simulink library "gnss_sdr_galileo_e1_tcp_connector_tracking_lib"  (Simulink 7.6)
settings: Solver=VariableStepDiscrete  StartTime=0.0  StopTime=10.0  RelTol=1e-3
undefined symbols (not defined in the file or in its folder): B_DLL, B_PLL, d_pdi_carr, d_pdi_code, k_DLL, k_PLL, magnitude, zeta_DLL, zeta_PLL
libraries: simulink x746, instrumentlib x2, dspindex x1
(part 5 of 5)

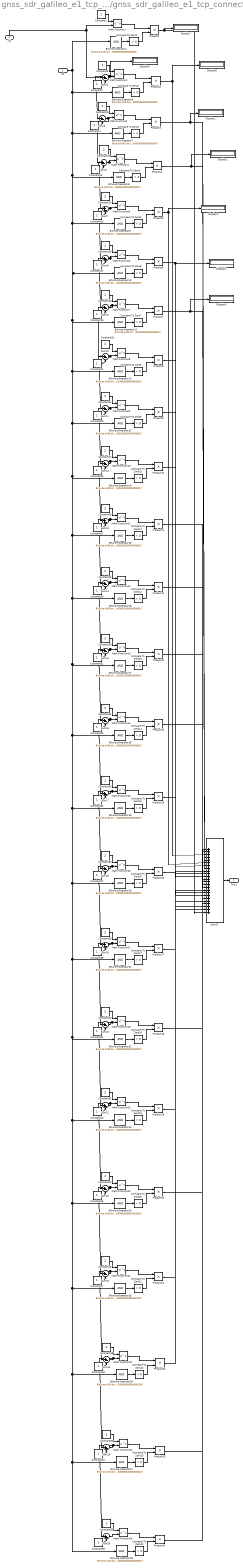
== system gnss_sdr_galileo_e1_tcp_connector_tracking_lib/gnss_sdr/gnss_sdr_galileo_e1_tcp_connector_tracking_rx/Subsystem6/hex2float/Subsystem ==
  In1 : Inport
  In2 : Inport  Port=2
  Bitwise Operator1 : simulink/Logic and Bit Operations/Bitwise Operator  logicop=AND  UseBitMask=on  BitMask=bin2dec('0100000000000000000000000')  BitMaskRealWorld=Stored Integer
  Bitwise Operator10 : simulink/Logic and Bit Operations/Bitwise Operator  logicop=AND  UseBitMask=on  BitMask=bin2dec('0000001000000000000000000')  BitMaskRealWorld=Stored Integer
  Bitwise Operator11 : simulink/Logic and Bit Operations/Bitwise Operator  logicop=AND  UseBitMask=on  BitMask=bin2dec('0000000100000000000000000')  BitMaskRealWorld=Stored Integer
  Bitwise Operator12 : simulink/Logic and Bit Operations/Bitwise Operator  logicop=AND  UseBitMask=on  BitMask=bin2dec('0000000010000000000000000')  BitMaskRealWorld=Stored Integer
  Bitwise Operator13 : simulink/Logic and Bit Operations/Bitwise Operator  logicop=AND  UseBitMask=on  BitMask=bin2dec('0000000001000000000000000')  BitMaskRealWorld=Stored Integer
  Bitwise Operator14 : simulink/Logic and Bit Operations/Bitwise Operator  logicop=AND  UseBitMask=on  BitMask=bin2dec('0000000000100000000000000')  BitMaskRealWorld=Stored Integer
  Bitwise Operator15 : simulink/Logic and Bit Operations/Bitwise Operator  logicop=AND  UseBitMask=on  BitMask=bin2dec('0000000000010000000000000')  BitMaskRealWorld=Stored Integer
  Bitwise Operator16 : simulink/Logic and Bit Operations/Bitwise Operator  logicop=AND  UseBitMask=on  BitMask=bin2dec('0000000000001000000000000')  BitMaskRealWorld=Stored Integer
  Bitwise Operator17 : simulink/Logic and Bit Operations/Bitwise Operator  logicop=AND  UseBitMask=on  BitMask=bin2dec('0000000000000100000000000')  BitMaskRealWorld=Stored Integer
  Bitwise Operator18 : simulink/Logic and Bit Operations/Bitwise Operator  logicop=AND  UseBitMask=on  BitMask=bin2dec('0000000000000010000000000')  BitMaskRealWorld=Stored Integer
  Bitwise Operator19 : simulink/Logic and Bit Operations/Bitwise Operator  logicop=AND  UseBitMask=on  BitMask=bin2dec('0000000000000001000000000')  BitMaskRealWorld=Stored Integer
  Bitwise Operator20 : simulink/Logic and Bit Operations/Bitwise Operator  logicop=AND  UseBitMask=on  BitMask=bin2dec('0000000000000000100000000')  BitMaskRealWorld=Stored Integer
  Bitwise Operator21 : simulink/Logic and Bit Operations/Bitwise Operator  logicop=AND  UseBitMask=on  BitMask=bin2dec('0000000000000000010000000')  BitMaskRealWorld=Stored Integer
  Bitwise Operator22 : simulink/Logic and Bit Operations/Bitwise Operator  logicop=AND  UseBitMask=on  BitMask=bin2dec('0000000000000000001000000')  BitMaskRealWorld=Stored Integer
  Bitwise Operator23 : simulink/Logic and Bit Operations/Bitwise Operator  logicop=AND  UseBitMask=on  BitMask=bin2dec('0000000000000000000100000')  BitMaskRealWorld=Stored Integer
  Bitwise Operator24 : simulink/Logic and Bit Operations/Bitwise Operator  logicop=AND  UseBitMask=on  BitMask=bin2dec('0000000000000000000010000')  BitMaskRealWorld=Stored Integer
  Bitwise Operator25 : simulink/Logic and Bit Operations/Bitwise Operator  logicop=AND  UseBitMask=on  BitMask=bin2dec('0000000000000000000001000')  BitMaskRealWorld=Stored Integer
  Bitwise Operator26 : simulink/Logic and Bit Operations/Bitwise Operator  logicop=AND  UseBitMask=on  BitMask=bin2dec('0000000000000000000000100')  BitMaskRealWorld=Stored Integer
  Bitwise Operator27 : simulink/Logic and Bit Operations/Bitwise Operator  logicop=AND  UseBitMask=on  BitMask=bin2dec('0000000000000000000000010')  BitMaskRealWorld=Stored Integer
  Bitwise Operator28 : simulink/Logic and Bit Operations/Bitwise Operator  logicop=AND  UseBitMask=on  BitMask=bin2dec('0000000000000000000000001')  BitMaskRealWorld=Stored Integer
  Bitwise Operator6 : simulink/Logic and Bit Operations/Bitwise Operator  logicop=AND  UseBitMask=on  BitMask=bin2dec('0010000000000000000000000')  BitMaskRealWorld=Stored Integer
  Bitwise Operator7 : simulink/Logic and Bit Operations/Bitwise Operator  logicop=AND  UseBitMask=on  BitMask=bin2dec('0001000000000000000000000')  BitMaskRealWorld=Stored Integer
  Bitwise Operator8 : simulink/Logic and Bit Operations/Bitwise Operator  logicop=AND  UseBitMask=on  BitMask=bin2dec('0000100000000000000000000')  BitMaskRealWorld=Stored Integer
  Bitwise Operator9 : simulink/Logic and Bit Operations/Bitwise Operator  logicop=AND  UseBitMask=on  BitMask=bin2dec('0000010000000000000000000')  BitMaskRealWorld=Stored Integer
  Compare To Zero{1..24} (24 alike) : simulink/Logic and Bit Operations/Compare To Zero  SystemSampleTime=-1  relop=>  LogicOutDataTypeMode=uint8  ZeroCross=off
  Constant{1,8,10,12,14,16,18,20,22,24,26,28,30,32,34,36,38,40,42,44,46,48,50,52} (24 alike) : Constant  Value=2
  Constant{2,11,13,15,17,19,21,23,25,27,29,31,33,35,37,39,41,43,45,47,49,51,53} (23 alike) : Constant
  Display{1..8} (8 alike) : Display
  Math Function{1..24} (24 alike) : Math  Operator=pow  SaturateOnIntegerOverflow=on
  Product{1..24} (24 alike) : Product  RndMeth=Zero
  Sum{1,5..26} (23 alike) : Sum  Inputs=|+-
  Sum27 : Sum  Inputs=|++++++++++++++++++++++++
  Out1 : Outport
  wires:
  Constant8/1 -> Math Function2/1
  Bitwise Operator6/1 -> Compare To Zero2/1
  Compare To Zero2/1 -> Product2/2
  Math Function2/1 -> Product2/1
  Constant10/1 -> Math Function3/1
  Bitwise Operator7/1 -> Compare To Zero3/1
  Compare To Zero3/1 -> Product3/2
  Math Function3/1 -> Product3/1
  Constant11/1 -> Sum5/2
  Sum5/1 -> Sum6/1, Math Function3/2
  Constant12/1 -> Math Function4/1
  Bitwise Operator8/1 -> Compare To Zero4/1
  Compare To Zero4/1 -> Product4/2
  Math Function4/1 -> Product4/1
  Constant13/1 -> Sum6/2
  Sum6/1 -> Sum7/1, Math Function4/2
  Constant14/1 -> Math Function5/1
  Bitwise Operator9/1 -> Compare To Zero5/1
  Compare To Zero5/1 -> Product5/2
  Math Function5/1 -> Product5/1
  Constant15/1 -> Sum7/2
  Sum7/1 -> Sum8/1, Math Function5/2
  Constant16/1 -> Math Function6/1
  Bitwise Operator10/1 -> Compare To Zero6/1
  Compare To Zero6/1 -> Product6/2
  Math Function6/1 -> Product6/1
  Constant17/1 -> Sum8/2
  Sum8/1 -> Sum9/1, Math Function6/2
  Constant18/1 -> Math Function7/1
  Bitwise Operator11/1 -> Compare To Zero7/1
  Compare To Zero7/1 -> Product7/2
  Math Function7/1 -> Product7/1
  Constant19/1 -> Sum9/2
  Sum9/1 -> Math Function7/2, Sum10/1
  Constant20/1 -> Math Function8/1
  Bitwise Operator12/1 -> Compare To Zero8/1
  Compare To Zero8/1 -> Product8/2
  Math Function8/1 -> Product8/1
  Constant21/1 -> Sum10/2
  Sum10/1 -> Math Function8/2, Sum11/1
  Constant22/1 -> Math Function9/1
  Bitwise Operator13/1 -> Compare To Zero9/1
  Compare To Zero9/1 -> Product9/2
  Math Function9/1 -> Product9/1
  Constant23/1 -> Sum11/2
  Sum11/1 -> Math Function9/2, Sum12/1
  Constant24/1 -> Math Function10/1
  Bitwise Operator14/1 -> Compare To Zero10/1
  Compare To Zero10/1 -> Product10/2
  Math Function10/1 -> Product10/1
  Constant25/1 -> Sum12/2
  Sum12/1 -> Math Function10/2, Sum13/1
  Constant26/1 -> Math Function11/1
  Bitwise Operator15/1 -> Compare To Zero11/1
  Compare To Zero11/1 -> Product11/2
  Math Function11/1 -> Product11/1
  Constant27/1 -> Sum13/2
  Sum13/1 -> Math Function11/2, Sum14/1
  Constant28/1 -> Math Function12/1
  Bitwise Operator16/1 -> Compare To Zero12/1
  Compare To Zero12/1 -> Product12/2
  Math Function12/1 -> Product12/1
  Constant29/1 -> Sum14/2
  Sum14/1 -> Math Function12/2, Sum15/1
  Constant30/1 -> Math Function13/1
  Bitwise Operator17/1 -> Compare To Zero13/1
  Compare To Zero13/1 -> Product13/2
  Math Function13/1 -> Product13/1
  Constant31/1 -> Sum15/2
  Sum15/1 -> Math Function13/2, Sum16/1
  Constant32/1 -> Math Function14/1
  Bitwise Operator18/1 -> Compare To Zero14/1
  Compare To Zero14/1 -> Product14/2
  Math Function14/1 -> Product14/1
  Constant33/1 -> Sum16/2
  Sum16/1 -> Math Function14/2, Sum17/1
  Constant34/1 -> Math Function15/1
  Bitwise Operator19/1 -> Compare To Zero15/1
  Compare To Zero15/1 -> Product15/2
  Math Function15/1 -> Product15/1
  Constant35/1 -> Sum17/2
  Sum17/1 -> Math Function15/2, Sum18/1
  Constant36/1 -> Math Function16/1
  Bitwise Operator20/1 -> Compare To Zero16/1
  Compare To Zero16/1 -> Product16/2
  Math Function16/1 -> Product16/1
  Constant37/1 -> Sum18/2
  Sum18/1 -> Math Function16/2, Sum19/1
  Constant38/1 -> Math Function17/1
  Bitwise Operator21/1 -> Compare To Zero17/1
  Compare To Zero17/1 -> Product17/2
  Math Function17/1 -> Product17/1
  Constant39/1 -> Sum19/2
  Sum19/1 -> Math Function17/2, Sum20/1
  Constant40/1 -> Math Function18/1
  Bitwise Operator22/1 -> Compare To Zero18/1
  Compare To Zero18/1 -> Product18/2
  Math Function18/1 -> Product18/1
  Constant41/1 -> Sum20/2
  Sum20/1 -> Math Function18/2, Sum21/1
  Constant42/1 -> Math Function19/1
  Bitwise Operator23/1 -> Compare To Zero19/1
  Compare To Zero19/1 -> Product19/2
  Math Function19/1 -> Product19/1
  Constant43/1 -> Sum21/2
  Sum21/1 -> Math Function19/2, Sum22/1
  Constant44/1 -> Math Function20/1
  Bitwise Operator24/1 -> Compare To Zero20/1
  Compare To Zero20/1 -> Product20/2
  Math Function20/1 -> Product20/1
  Constant45/1 -> Sum22/2
  Sum22/1 -> Math Function20/2, Sum23/1
  Constant46/1 -> Math Function21/1
  Bitwise Operator25/1 -> Compare To Zero21/1
  Compare To Zero21/1 -> Product21/2
  Math Function21/1 -> Product21/1
  Constant47/1 -> Sum23/2
  Sum23/1 -> Math Function21/2, Sum24/1
  Constant48/1 -> Math Function22/1
  Bitwise Operator26/1 -> Compare To Zero22/1
  Compare To Zero22/1 -> Product22/2
  Math Function22/1 -> Product22/1
  Constant49/1 -> Sum24/2
  Sum24/1 -> Math Function22/2, Sum25/1
  Constant50/1 -> Math Function23/1
  Bitwise Operator27/1 -> Compare To Zero23/1
  Compare To Zero23/1 -> Product23/2
  Math Function23/1 -> Product23/1
  Constant51/1 -> Sum25/2
  Sum25/1 -> Math Function23/2, Sum26/1
  Constant52/1 -> Math Function24/1
  Bitwise Operator28/1 -> Compare To Zero24/1
  Compare To Zero24/1 -> Product24/2
  Math Function24/1 -> Product24/1
  Constant53/1 -> Sum26/2
  Sum26/1 -> Math Function24/2
  Product2/1 -> Sum27/3, Display5/1
  Product3/1 -> Sum27/4, Display1/1
  Product4/1 -> Sum27/5, Display2/1
  Product5/1 -> Sum27/6, Display3/1
  Product6/1 -> Sum27/7, Display4/1
  Product7/1 -> Sum27/8, Display6/1
  Product8/1 -> Sum27/9
  Product9/1 -> Sum27/10
  Product10/1 -> Sum27/11
  Product11/1 -> Sum27/12
  Product12/1 -> Sum27/13
  Product13/1 -> Sum27/14
  Product14/1 -> Sum27/15
  Product15/1 -> Sum27/16
  Product16/1 -> Sum27/17
  Product17/1 -> Sum27/18
  Product18/1 -> Sum27/19
  Product19/1 -> Sum27/20
  Product20/1 -> Sum27/21
  Product21/1 -> Sum27/22
  Product22/1 -> Sum27/23
  Product23/1 -> Sum27/2
  Product24/1 -> Sum27/1
  In1/1 -> Math Function1/2, Sum1/1
  In2/1 -> Bitwise Operator6/1, Bitwise Operator7/1, Bitwise Operator8/1, Bitwise Operator9/1, Bitwise Operator10/1, Bitwise Operator11/1, Bitwise Operator12/1, Bitwise Operator13/1, Bitwise Operator14/1, Bitwise Operator15/1, Bitwise Operator16/1, Bitwise Operator17/1, Bitwise Operator18/1, Bitwise Operator19/1, Bitwise Operator20/1, Bitwise Operator21/1, Bitwise Operator22/1, Bitwise Operator23/1, Bitwise Operator24/1, Bitwise Operator25/1, Bitwise Operator26/1, Bitwise Operator27/1, Bitwise Operator28/1, Bitwise Operator1/1
  Sum27/1 -> Out1/1
  Constant1/1 -> Math Function1/1
  Bitwise Operator1/1 -> Compare To Zero1/1
  Compare To Zero1/1 -> Product1/2
  Math Function1/1 -> Product1/1
  Constant2/1 -> Sum1/2
  Sum1/1 -> Math Function2/2, Display8/1, Sum5/1
  Product1/1 -> Display7/1, Sum27/24

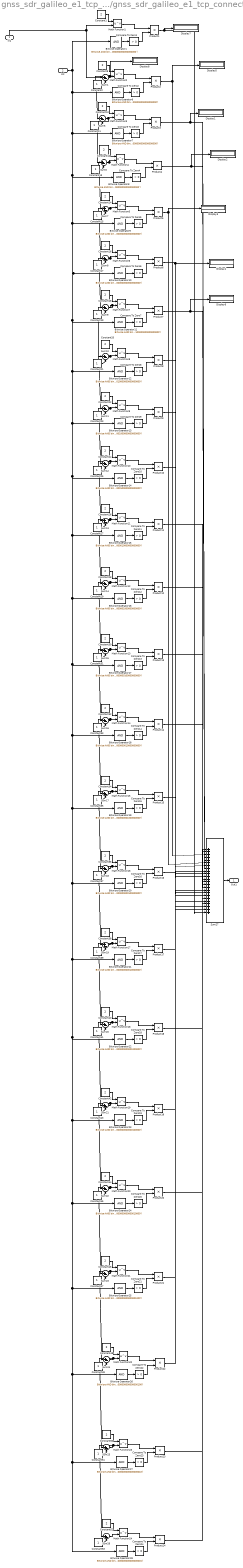
== system gnss_sdr_galileo_e1_tcp_connector_tracking_lib/gnss_sdr/gnss_sdr_galileo_e1_tcp_connector_tracking_rx/Subsystem7/hex2float/Subsystem ==
  In1 : Inport
  In2 : Inport  Port=2
  Bitwise Operator1 : simulink/Logic and Bit Operations/Bitwise Operator  logicop=AND  UseBitMask=on  BitMask=bin2dec('0100000000000000000000000')  BitMaskRealWorld=Stored Integer
  Bitwise Operator10 : simulink/Logic and Bit Operations/Bitwise Operator  logicop=AND  UseBitMask=on  BitMask=bin2dec('0000001000000000000000000')  BitMaskRealWorld=Stored Integer
  Bitwise Operator11 : simulink/Logic and Bit Operations/Bitwise Operator  logicop=AND  UseBitMask=on  BitMask=bin2dec('0000000100000000000000000')  BitMaskRealWorld=Stored Integer
  Bitwise Operator12 : simulink/Logic and Bit Operations/Bitwise Operator  logicop=AND  UseBitMask=on  BitMask=bin2dec('0000000010000000000000000')  BitMaskRealWorld=Stored Integer
  Bitwise Operator13 : simulink/Logic and Bit Operations/Bitwise Operator  logicop=AND  UseBitMask=on  BitMask=bin2dec('0000000001000000000000000')  BitMaskRealWorld=Stored Integer
  Bitwise Operator14 : simulink/Logic and Bit Operations/Bitwise Operator  logicop=AND  UseBitMask=on  BitMask=bin2dec('0000000000100000000000000')  BitMaskRealWorld=Stored Integer
  Bitwise Operator15 : simulink/Logic and Bit Operations/Bitwise Operator  logicop=AND  UseBitMask=on  BitMask=bin2dec('0000000000010000000000000')  BitMaskRealWorld=Stored Integer
  Bitwise Operator16 : simulink/Logic and Bit Operations/Bitwise Operator  logicop=AND  UseBitMask=on  BitMask=bin2dec('0000000000001000000000000')  BitMaskRealWorld=Stored Integer
  Bitwise Operator17 : simulink/Logic and Bit Operations/Bitwise Operator  logicop=AND  UseBitMask=on  BitMask=bin2dec('0000000000000100000000000')  BitMaskRealWorld=Stored Integer
  Bitwise Operator18 : simulink/Logic and Bit Operations/Bitwise Operator  logicop=AND  UseBitMask=on  BitMask=bin2dec('0000000000000010000000000')  BitMaskRealWorld=Stored Integer
  Bitwise Operator19 : simulink/Logic and Bit Operations/Bitwise Operator  logicop=AND  UseBitMask=on  BitMask=bin2dec('0000000000000001000000000')  BitMaskRealWorld=Stored Integer
  Bitwise Operator20 : simulink/Logic and Bit Operations/Bitwise Operator  logicop=AND  UseBitMask=on  BitMask=bin2dec('0000000000000000100000000')  BitMaskRealWorld=Stored Integer
  Bitwise Operator21 : simulink/Logic and Bit Operations/Bitwise Operator  logicop=AND  UseBitMask=on  BitMask=bin2dec('0000000000000000010000000')  BitMaskRealWorld=Stored Integer
  Bitwise Operator22 : simulink/Logic and Bit Operations/Bitwise Operator  logicop=AND  UseBitMask=on  BitMask=bin2dec('0000000000000000001000000')  BitMaskRealWorld=Stored Integer
  Bitwise Operator23 : simulink/Logic and Bit Operations/Bitwise Operator  logicop=AND  UseBitMask=on  BitMask=bin2dec('0000000000000000000100000')  BitMaskRealWorld=Stored Integer
  Bitwise Operator24 : simulink/Logic and Bit Operations/Bitwise Operator  logicop=AND  UseBitMask=on  BitMask=bin2dec('0000000000000000000010000')  BitMaskRealWorld=Stored Integer
  Bitwise Operator25 : simulink/Logic and Bit Operations/Bitwise Operator  logicop=AND  UseBitMask=on  BitMask=bin2dec('0000000000000000000001000')  BitMaskRealWorld=Stored Integer
  Bitwise Operator26 : simulink/Logic and Bit Operations/Bitwise Operator  logicop=AND  UseBitMask=on  BitMask=bin2dec('0000000000000000000000100')  BitMaskRealWorld=Stored Integer
  Bitwise Operator27 : simulink/Logic and Bit Operations/Bitwise Operator  logicop=AND  UseBitMask=on  BitMask=bin2dec('0000000000000000000000010')  BitMaskRealWorld=Stored Integer
  Bitwise Operator28 : simulink/Logic and Bit Operations/Bitwise Operator  logicop=AND  UseBitMask=on  BitMask=bin2dec('0000000000000000000000001')  BitMaskRealWorld=Stored Integer
  Bitwise Operator6 : simulink/Logic and Bit Operations/Bitwise Operator  logicop=AND  UseBitMask=on  BitMask=bin2dec('0010000000000000000000000')  BitMaskRealWorld=Stored Integer
  Bitwise Operator7 : simulink/Logic and Bit Operations/Bitwise Operator  logicop=AND  UseBitMask=on  BitMask=bin2dec('0001000000000000000000000')  BitMaskRealWorld=Stored Integer
  Bitwise Operator8 : simulink/Logic and Bit Operations/Bitwise Operator  logicop=AND  UseBitMask=on  BitMask=bin2dec('0000100000000000000000000')  BitMaskRealWorld=Stored Integer
  Bitwise Operator9 : simulink/Logic and Bit Operations/Bitwise Operator  logicop=AND  UseBitMask=on  BitMask=bin2dec('0000010000000000000000000')  BitMaskRealWorld=Stored Integer
  Compare To Zero{1..24} (24 alike) : simulink/Logic and Bit Operations/Compare To Zero  SystemSampleTime=-1  relop=>  LogicOutDataTypeMode=uint8  ZeroCross=off
  Constant{1,8,10,12,14,16,18,20,22,24,26,28,30,32,34,36,38,40,42,44,46,48,50,52} (24 alike) : Constant  Value=2
  Constant{2,11,13,15,17,19,21,23,25,27,29,31,33,35,37,39,41,43,45,47,49,51,53} (23 alike) : Constant
  Display{1..8} (8 alike) : Display
  Math Function{1..24} (24 alike) : Math  Operator=pow  SaturateOnIntegerOverflow=on
  Product{1..24} (24 alike) : Product  RndMeth=Zero
  Sum{1,5..26} (23 alike) : Sum  Inputs=|+-
  Sum27 : Sum  Inputs=|++++++++++++++++++++++++
  Out1 : Outport
  wires:
  Product1/1 -> Sum27/24, Display7/1
  Sum1/1 -> Sum5/1, Display8/1, Math Function2/2
  Constant2/1 -> Sum1/2
  Math Function1/1 -> Product1/1
  Compare To Zero1/1 -> Product1/2
  Bitwise Operator1/1 -> Compare To Zero1/1
  Constant1/1 -> Math Function1/1
  Sum27/1 -> Out1/1
  In2/1 -> Bitwise Operator1/1, Bitwise Operator28/1, Bitwise Operator27/1, Bitwise Operator26/1, Bitwise Operator25/1, Bitwise Operator24/1, Bitwise Operator23/1, Bitwise Operator22/1, Bitwise Operator21/1, Bitwise Operator20/1, Bitwise Operator19/1, Bitwise Operator18/1, Bitwise Operator17/1, Bitwise Operator16/1, Bitwise Operator15/1, Bitwise Operator14/1, Bitwise Operator13/1, Bitwise Operator12/1, Bitwise Operator11/1, Bitwise Operator10/1, Bitwise Operator9/1, Bitwise Operator8/1, Bitwise Operator7/1, Bitwise Operator6/1
  In1/1 -> Sum1/1, Math Function1/2
  Product24/1 -> Sum27/1
  Product23/1 -> Sum27/2
  Product22/1 -> Sum27/23
  Product21/1 -> Sum27/22
  Product20/1 -> Sum27/21
  Product19/1 -> Sum27/20
  Product18/1 -> Sum27/19
  Product17/1 -> Sum27/18
  Product16/1 -> Sum27/17
  Product15/1 -> Sum27/16
  Product14/1 -> Sum27/15
  Product13/1 -> Sum27/14
  Product12/1 -> Sum27/13
  Product11/1 -> Sum27/12
  Product10/1 -> Sum27/11
  Product9/1 -> Sum27/10
  Product8/1 -> Sum27/9
  Product7/1 -> Display6/1, Sum27/8
  Product6/1 -> Display4/1, Sum27/7
  Product5/1 -> Display3/1, Sum27/6
  Product4/1 -> Display2/1, Sum27/5
  Product3/1 -> Display1/1, Sum27/4
  Product2/1 -> Display5/1, Sum27/3
  Sum26/1 -> Math Function24/2
  Constant53/1 -> Sum26/2
  Math Function24/1 -> Product24/1
  Compare To Zero24/1 -> Product24/2
  Bitwise Operator28/1 -> Compare To Zero24/1
  Constant52/1 -> Math Function24/1
  Sum25/1 -> Sum26/1, Math Function23/2
  Constant51/1 -> Sum25/2
  Math Function23/1 -> Product23/1
  Compare To Zero23/1 -> Product23/2
  Bitwise Operator27/1 -> Compare To Zero23/1
  Constant50/1 -> Math Function23/1
  Sum24/1 -> Sum25/1, Math Function22/2
  Constant49/1 -> Sum24/2
  Math Function22/1 -> Product22/1
  Compare To Zero22/1 -> Product22/2
  Bitwise Operator26/1 -> Compare To Zero22/1
  Constant48/1 -> Math Function22/1
  Sum23/1 -> Sum24/1, Math Function21/2
  Constant47/1 -> Sum23/2
  Math Function21/1 -> Product21/1
  Compare To Zero21/1 -> Product21/2
  Bitwise Operator25/1 -> Compare To Zero21/1
  Constant46/1 -> Math Function21/1
  Sum22/1 -> Sum23/1, Math Function20/2
  Constant45/1 -> Sum22/2
  Math Function20/1 -> Product20/1
  Compare To Zero20/1 -> Product20/2
  Bitwise Operator24/1 -> Compare To Zero20/1
  Constant44/1 -> Math Function20/1
  Sum21/1 -> Sum22/1, Math Function19/2
  Constant43/1 -> Sum21/2
  Math Function19/1 -> Product19/1
  Compare To Zero19/1 -> Product19/2
  Bitwise Operator23/1 -> Compare To Zero19/1
  Constant42/1 -> Math Function19/1
  Sum20/1 -> Sum21/1, Math Function18/2
  Constant41/1 -> Sum20/2
  Math Function18/1 -> Product18/1
  Compare To Zero18/1 -> Product18/2
  Bitwise Operator22/1 -> Compare To Zero18/1
  Constant40/1 -> Math Function18/1
  Sum19/1 -> Sum20/1, Math Function17/2
  Constant39/1 -> Sum19/2
  Math Function17/1 -> Product17/1
  Compare To Zero17/1 -> Product17/2
  Bitwise Operator21/1 -> Compare To Zero17/1
  Constant38/1 -> Math Function17/1
  Sum18/1 -> Sum19/1, Math Function16/2
  Constant37/1 -> Sum18/2
  Math Function16/1 -> Product16/1
  Compare To Zero16/1 -> Product16/2
  Bitwise Operator20/1 -> Compare To Zero16/1
  Constant36/1 -> Math Function16/1
  Sum17/1 -> Sum18/1, Math Function15/2
  Constant35/1 -> Sum17/2
  Math Function15/1 -> Product15/1
  Compare To Zero15/1 -> Product15/2
  Bitwise Operator19/1 -> Compare To Zero15/1
  Constant34/1 -> Math Function15/1
  Sum16/1 -> Sum17/1, Math Function14/2
  Constant33/1 -> Sum16/2
  Math Function14/1 -> Product14/1
  Compare To Zero14/1 -> Product14/2
  Bitwise Operator18/1 -> Compare To Zero14/1
  Constant32/1 -> Math Function14/1
  Sum15/1 -> Sum16/1, Math Function13/2
  Constant31/1 -> Sum15/2
  Math Function13/1 -> Product13/1
  Compare To Zero13/1 -> Product13/2
  Bitwise Operator17/1 -> Compare To Zero13/1
  Constant30/1 -> Math Function13/1
  Sum14/1 -> Sum15/1, Math Function12/2
  Constant29/1 -> Sum14/2
  Math Function12/1 -> Product12/1
  Compare To Zero12/1 -> Product12/2
  Bitwise Operator16/1 -> Compare To Zero12/1
  Constant28/1 -> Math Function12/1
  Sum13/1 -> Sum14/1, Math Function11/2
  Constant27/1 -> Sum13/2
  Math Function11/1 -> Product11/1
  Compare To Zero11/1 -> Product11/2
  Bitwise Operator15/1 -> Compare To Zero11/1
  Constant26/1 -> Math Function11/1
  Sum12/1 -> Sum13/1, Math Function10/2
  Constant25/1 -> Sum12/2
  Math Function10/1 -> Product10/1
  Compare To Zero10/1 -> Product10/2
  Bitwise Operator14/1 -> Compare To Zero10/1
  Constant24/1 -> Math Function10/1
  Sum11/1 -> Sum12/1, Math Function9/2
  Constant23/1 -> Sum11/2
  Math Function9/1 -> Product9/1
  Compare To Zero9/1 -> Product9/2
  Bitwise Operator13/1 -> Compare To Zero9/1
  Constant22/1 -> Math Function9/1
  Sum10/1 -> Sum11/1, Math Function8/2
  Constant21/1 -> Sum10/2
  Math Function8/1 -> Product8/1
  Compare To Zero8/1 -> Product8/2
  Bitwise Operator12/1 -> Compare To Zero8/1
  Constant20/1 -> Math Function8/1
  Sum9/1 -> Sum10/1, Math Function7/2
  Constant19/1 -> Sum9/2
  Math Function7/1 -> Product7/1
  Compare To Zero7/1 -> Product7/2
  Bitwise Operator11/1 -> Compare To Zero7/1
  Constant18/1 -> Math Function7/1
  Sum8/1 -> Math Function6/2, Sum9/1
  Constant17/1 -> Sum8/2
  Math Function6/1 -> Product6/1
  Compare To Zero6/1 -> Product6/2
  Bitwise Operator10/1 -> Compare To Zero6/1
  Constant16/1 -> Math Function6/1
  Sum7/1 -> Math Function5/2, Sum8/1
  Constant15/1 -> Sum7/2
  Math Function5/1 -> Product5/1
  Compare To Zero5/1 -> Product5/2
  Bitwise Operator9/1 -> Compare To Zero5/1
  Constant14/1 -> Math Function5/1
  Sum6/1 -> Math Function4/2, Sum7/1
  Constant13/1 -> Sum6/2
  Math Function4/1 -> Product4/1
  Compare To Zero4/1 -> Product4/2
  Bitwise Operator8/1 -> Compare To Zero4/1
  Constant12/1 -> Math Function4/1
  Sum5/1 -> Math Function3/2, Sum6/1
  Constant11/1 -> Sum5/2
  Math Function3/1 -> Product3/1
  Compare To Zero3/1 -> Product3/2
  Bitwise Operator7/1 -> Compare To Zero3/1
  Constant10/1 -> Math Function3/1
  Math Function2/1 -> Product2/1
  Compare To Zero2/1 -> Product2/2
  Bitwise Operator6/1 -> Compare To Zero2/1
  Constant8/1 -> Math Function2/1

== system gnss_sdr_galileo_e1_tcp_connector_tracking_lib/gnss_sdr/gnss_sdr_galileo_e1_tcp_connector_tracking_rx/Subsystem8/hex2float/Subsystem ==
  In1 : Inport
  In2 : Inport  Port=2
  Bitwise Operator1 : simulink/Logic and Bit Operations/Bitwise Operator  logicop=AND  UseBitMask=on  BitMask=bin2dec('0100000000000000000000000')  BitMaskRealWorld=Stored Integer
  Bitwise Operator10 : simulink/Logic and Bit Operations/Bitwise Operator  logicop=AND  UseBitMask=on  BitMask=bin2dec('0000001000000000000000000')  BitMaskRealWorld=Stored Integer
  Bitwise Operator11 : simulink/Logic and Bit Operations/Bitwise Operator  logicop=AND  UseBitMask=on  BitMask=bin2dec('0000000100000000000000000')  BitMaskRealWorld=Stored Integer
  Bitwise Operator12 : simulink/Logic and Bit Operations/Bitwise Operator  logicop=AND  UseBitMask=on  BitMask=bin2dec('0000000010000000000000000')  BitMaskRealWorld=Stored Integer
  Bitwise Operator13 : simulink/Logic and Bit Operations/Bitwise Operator  logicop=AND  UseBitMask=on  BitMask=bin2dec('0000000001000000000000000')  BitMaskRealWorld=Stored Integer
  Bitwise Operator14 : simulink/Logic and Bit Operations/Bitwise Operator  logicop=AND  UseBitMask=on  BitMask=bin2dec('0000000000100000000000000')  BitMaskRealWorld=Stored Integer
  Bitwise Operator15 : simulink/Logic and Bit Operations/Bitwise Operator  logicop=AND  UseBitMask=on  BitMask=bin2dec('0000000000010000000000000')  BitMaskRealWorld=Stored Integer
  Bitwise Operator16 : simulink/Logic and Bit Operations/Bitwise Operator  logicop=AND  UseBitMask=on  BitMask=bin2dec('0000000000001000000000000')  BitMaskRealWorld=Stored Integer
  Bitwise Operator17 : simulink/Logic and Bit Operations/Bitwise Operator  logicop=AND  UseBitMask=on  BitMask=bin2dec('0000000000000100000000000')  BitMaskRealWorld=Stored Integer
  Bitwise Operator18 : simulink/Logic and Bit Operations/Bitwise Operator  logicop=AND  UseBitMask=on  BitMask=bin2dec('0000000000000010000000000')  BitMaskRealWorld=Stored Integer
  Bitwise Operator19 : simulink/Logic and Bit Operations/Bitwise Operator  logicop=AND  UseBitMask=on  BitMask=bin2dec('0000000000000001000000000')  BitMaskRealWorld=Stored Integer
  Bitwise Operator20 : simulink/Logic and Bit Operations/Bitwise Operator  logicop=AND  UseBitMask=on  BitMask=bin2dec('0000000000000000100000000')  BitMaskRealWorld=Stored Integer
  Bitwise Operator21 : simulink/Logic and Bit Operations/Bitwise Operator  logicop=AND  UseBitMask=on  BitMask=bin2dec('0000000000000000010000000')  BitMaskRealWorld=Stored Integer
  Bitwise Operator22 : simulink/Logic and Bit Operations/Bitwise Operator  logicop=AND  UseBitMask=on  BitMask=bin2dec('0000000000000000001000000')  BitMaskRealWorld=Stored Integer
  Bitwise Operator23 : simulink/Logic and Bit Operations/Bitwise Operator  logicop=AND  UseBitMask=on  BitMask=bin2dec('0000000000000000000100000')  BitMaskRealWorld=Stored Integer
  Bitwise Operator24 : simulink/Logic and Bit Operations/Bitwise Operator  logicop=AND  UseBitMask=on  BitMask=bin2dec('0000000000000000000010000')  BitMaskRealWorld=Stored Integer
  Bitwise Operator25 : simulink/Logic and Bit Operations/Bitwise Operator  logicop=AND  UseBitMask=on  BitMask=bin2dec('0000000000000000000001000')  BitMaskRealWorld=Stored Integer
  Bitwise Operator26 : simulink/Logic and Bit Operations/Bitwise Operator  logicop=AND  UseBitMask=on  BitMask=bin2dec('0000000000000000000000100')  BitMaskRealWorld=Stored Integer
  Bitwise Operator27 : simulink/Logic and Bit Operations/Bitwise Operator  logicop=AND  UseBitMask=on  BitMask=bin2dec('0000000000000000000000010')  BitMaskRealWorld=Stored Integer
  Bitwise Operator28 : simulink/Logic and Bit Operations/Bitwise Operator  logicop=AND  UseBitMask=on  BitMask=bin2dec('0000000000000000000000001')  BitMaskRealWorld=Stored Integer
  Bitwise Operator6 : simulink/Logic and Bit Operations/Bitwise Operator  logicop=AND  UseBitMask=on  BitMask=bin2dec('0010000000000000000000000')  BitMaskRealWorld=Stored Integer
  Bitwise Operator7 : simulink/Logic and Bit Operations/Bitwise Operator  logicop=AND  UseBitMask=on  BitMask=bin2dec('0001000000000000000000000')  BitMaskRealWorld=Stored Integer
  Bitwise Operator8 : simulink/Logic and Bit Operations/Bitwise Operator  logicop=AND  UseBitMask=on  BitMask=bin2dec('0000100000000000000000000')  BitMaskRealWorld=Stored Integer
  Bitwise Operator9 : simulink/Logic and Bit Operations/Bitwise Operator  logicop=AND  UseBitMask=on  BitMask=bin2dec('0000010000000000000000000')  BitMaskRealWorld=Stored Integer
  Compare To Zero{1..24} (24 alike) : simulink/Logic and Bit Operations/Compare To Zero  SystemSampleTime=-1  relop=>  LogicOutDataTypeMode=uint8  ZeroCross=off
  Constant{1,8,10,12,14,16,18,20,22,24,26,28,30,32,34,36,38,40,42,44,46,48,50,52} (24 alike) : Constant  Value=2
  Constant{2,11,13,15,17,19,21,23,25,27,29,31,33,35,37,39,41,43,45,47,49,51,53} (23 alike) : Constant
  Display{1..8} (8 alike) : Display
  Math Function{1..24} (24 alike) : Math  Operator=pow  SaturateOnIntegerOverflow=on
  Product{1..24} (24 alike) : Product  RndMeth=Zero
  Sum{1,5..26} (23 alike) : Sum  Inputs=|+-
  Sum27 : Sum  Inputs=|++++++++++++++++++++++++
  Out1 : Outport
  wires:
  Product1/1 -> Sum27/24, Display7/1
  Sum1/1 -> Sum5/1, Display8/1, Math Function2/2
  Constant2/1 -> Sum1/2
  Math Function1/1 -> Product1/1
  Compare To Zero1/1 -> Product1/2
  Bitwise Operator1/1 -> Compare To Zero1/1
  Constant1/1 -> Math Function1/1
  Sum27/1 -> Out1/1
  In2/1 -> Bitwise Operator1/1, Bitwise Operator28/1, Bitwise Operator27/1, Bitwise Operator26/1, Bitwise Operator25/1, Bitwise Operator24/1, Bitwise Operator23/1, Bitwise Operator22/1, Bitwise Operator21/1, Bitwise Operator20/1, Bitwise Operator19/1, Bitwise Operator18/1, Bitwise Operator17/1, Bitwise Operator16/1, Bitwise Operator15/1, Bitwise Operator14/1, Bitwise Operator13/1, Bitwise Operator12/1, Bitwise Operator11/1, Bitwise Operator10/1, Bitwise Operator9/1, Bitwise Operator8/1, Bitwise Operator7/1, Bitwise Operator6/1
  In1/1 -> Sum1/1, Math Function1/2
  Product24/1 -> Sum27/1
  Product23/1 -> Sum27/2
  Product22/1 -> Sum27/23
  Product21/1 -> Sum27/22
  Product20/1 -> Sum27/21
  Product19/1 -> Sum27/20
  Product18/1 -> Sum27/19
  Product17/1 -> Sum27/18
  Product16/1 -> Sum27/17
  Product15/1 -> Sum27/16
  Product14/1 -> Sum27/15
  Product13/1 -> Sum27/14
  Product12/1 -> Sum27/13
  Product11/1 -> Sum27/12
  Product10/1 -> Sum27/11
  Product9/1 -> Sum27/10
  Product8/1 -> Sum27/9
  Product7/1 -> Display6/1, Sum27/8
  Product6/1 -> Display4/1, Sum27/7
  Product5/1 -> Display3/1, Sum27/6
  Product4/1 -> Display2/1, Sum27/5
  Product3/1 -> Display1/1, Sum27/4
  Product2/1 -> Display5/1, Sum27/3
  Sum26/1 -> Math Function24/2
  Constant53/1 -> Sum26/2
  Math Function24/1 -> Product24/1
  Compare To Zero24/1 -> Product24/2
  Bitwise Operator28/1 -> Compare To Zero24/1
  Constant52/1 -> Math Function24/1
  Sum25/1 -> Sum26/1, Math Function23/2
  Constant51/1 -> Sum25/2
  Math Function23/1 -> Product23/1
  Compare To Zero23/1 -> Product23/2
  Bitwise Operator27/1 -> Compare To Zero23/1
  Constant50/1 -> Math Function23/1
  Sum24/1 -> Sum25/1, Math Function22/2
  Constant49/1 -> Sum24/2
  Math Function22/1 -> Product22/1
  Compare To Zero22/1 -> Product22/2
  Bitwise Operator26/1 -> Compare To Zero22/1
  Constant48/1 -> Math Function22/1
  Sum23/1 -> Sum24/1, Math Function21/2
  Constant47/1 -> Sum23/2
  Math Function21/1 -> Product21/1
  Compare To Zero21/1 -> Product21/2
  Bitwise Operator25/1 -> Compare To Zero21/1
  Constant46/1 -> Math Function21/1
  Sum22/1 -> Sum23/1, Math Function20/2
  Constant45/1 -> Sum22/2
  Math Function20/1 -> Product20/1
  Compare To Zero20/1 -> Product20/2
  Bitwise Operator24/1 -> Compare To Zero20/1
  Constant44/1 -> Math Function20/1
  Sum21/1 -> Sum22/1, Math Function19/2
  Constant43/1 -> Sum21/2
  Math Function19/1 -> Product19/1
  Compare To Zero19/1 -> Product19/2
  Bitwise Operator23/1 -> Compare To Zero19/1
  Constant42/1 -> Math Function19/1
  Sum20/1 -> Sum21/1, Math Function18/2
  Constant41/1 -> Sum20/2
  Math Function18/1 -> Product18/1
  Compare To Zero18/1 -> Product18/2
  Bitwise Operator22/1 -> Compare To Zero18/1
  Constant40/1 -> Math Function18/1
  Sum19/1 -> Sum20/1, Math Function17/2
  Constant39/1 -> Sum19/2
  Math Function17/1 -> Product17/1
  Compare To Zero17/1 -> Product17/2
  Bitwise Operator21/1 -> Compare To Zero17/1
  Constant38/1 -> Math Function17/1
  Sum18/1 -> Sum19/1, Math Function16/2
  Constant37/1 -> Sum18/2
  Math Function16/1 -> Product16/1
  Compare To Zero16/1 -> Product16/2
  Bitwise Operator20/1 -> Compare To Zero16/1
  Constant36/1 -> Math Function16/1
  Sum17/1 -> Sum18/1, Math Function15/2
  Constant35/1 -> Sum17/2
  Math Function15/1 -> Product15/1
  Compare To Zero15/1 -> Product15/2
  Bitwise Operator19/1 -> Compare To Zero15/1
  Constant34/1 -> Math Function15/1
  Sum16/1 -> Sum17/1, Math Function14/2
  Constant33/1 -> Sum16/2
  Math Function14/1 -> Product14/1
  Compare To Zero14/1 -> Product14/2
  Bitwise Operator18/1 -> Compare To Zero14/1
  Constant32/1 -> Math Function14/1
  Sum15/1 -> Sum16/1, Math Function13/2
  Constant31/1 -> Sum15/2
  Math Function13/1 -> Product13/1
  Compare To Zero13/1 -> Product13/2
  Bitwise Operator17/1 -> Compare To Zero13/1
  Constant30/1 -> Math Function13/1
  Sum14/1 -> Sum15/1, Math Function12/2
  Constant29/1 -> Sum14/2
  Math Function12/1 -> Product12/1
  Compare To Zero12/1 -> Product12/2
  Bitwise Operator16/1 -> Compare To Zero12/1
  Constant28/1 -> Math Function12/1
  Sum13/1 -> Sum14/1, Math Function11/2
  Constant27/1 -> Sum13/2
  Math Function11/1 -> Product11/1
  Compare To Zero11/1 -> Product11/2
  Bitwise Operator15/1 -> Compare To Zero11/1
  Constant26/1 -> Math Function11/1
  Sum12/1 -> Sum13/1, Math Function10/2
  Constant25/1 -> Sum12/2
  Math Function10/1 -> Product10/1
  Compare To Zero10/1 -> Product10/2
  Bitwise Operator14/1 -> Compare To Zero10/1
  Constant24/1 -> Math Function10/1
  Sum11/1 -> Sum12/1, Math Function9/2
  Constant23/1 -> Sum11/2
  Math Function9/1 -> Product9/1
  Compare To Zero9/1 -> Product9/2
  Bitwise Operator13/1 -> Compare To Zero9/1
  Constant22/1 -> Math Function9/1
  Sum10/1 -> Sum11/1, Math Function8/2
  Constant21/1 -> Sum10/2
  Math Function8/1 -> Product8/1
  Compare To Zero8/1 -> Product8/2
  Bitwise Operator12/1 -> Compare To Zero8/1
  Constant20/1 -> Math Function8/1
  Sum9/1 -> Sum10/1, Math Function7/2
  Constant19/1 -> Sum9/2
  Math Function7/1 -> Product7/1
  Compare To Zero7/1 -> Product7/2
  Bitwise Operator11/1 -> Compare To Zero7/1
  Constant18/1 -> Math Function7/1
  Sum8/1 -> Math Function6/2, Sum9/1
  Constant17/1 -> Sum8/2
  Math Function6/1 -> Product6/1
  Compare To Zero6/1 -> Product6/2
  Bitwise Operator10/1 -> Compare To Zero6/1
  Constant16/1 -> Math Function6/1
  Sum7/1 -> Math Function5/2, Sum8/1
  Constant15/1 -> Sum7/2
  Math Function5/1 -> Product5/1
  Compare To Zero5/1 -> Product5/2
  Bitwise Operator9/1 -> Compare To Zero5/1
  Constant14/1 -> Math Function5/1
  Sum6/1 -> Math Function4/2, Sum7/1
  Constant13/1 -> Sum6/2
  Math Function4/1 -> Product4/1
  Compare To Zero4/1 -> Product4/2
  Bitwise Operator8/1 -> Compare To Zero4/1
  Constant12/1 -> Math Function4/1
  Sum5/1 -> Math Function3/2, Sum6/1
  Constant11/1 -> Sum5/2
  Math Function3/1 -> Product3/1
  Compare To Zero3/1 -> Product3/2
  Bitwise Operator7/1 -> Compare To Zero3/1
  Constant10/1 -> Math Function3/1
  Math Function2/1 -> Product2/1
  Compare To Zero2/1 -> Product2/2
  Bitwise Operator6/1 -> Compare To Zero2/1
  Constant8/1 -> Math Function2/1

== system gnss_sdr_galileo_e1_tcp_connector_tracking_lib/gnss_sdr/gnss_sdr_galileo_e1_tcp_connector_tracking_rx/Subsystem9/hex2float/Subsystem ==
  In1 : Inport
  In2 : Inport  Port=2
  Bitwise Operator1 : simulink/Logic and Bit Operations/Bitwise Operator  logicop=AND  UseBitMask=on  BitMask=bin2dec('0100000000000000000000000')  BitMaskRealWorld=Stored Integer
  Bitwise Operator10 : simulink/Logic and Bit Operations/Bitwise Operator  logicop=AND  UseBitMask=on  BitMask=bin2dec('0000001000000000000000000')  BitMaskRealWorld=Stored Integer
  Bitwise Operator11 : simulink/Logic and Bit Operations/Bitwise Operator  logicop=AND  UseBitMask=on  BitMask=bin2dec('0000000100000000000000000')  BitMaskRealWorld=Stored Integer
  Bitwise Operator12 : simulink/Logic and Bit Operations/Bitwise Operator  logicop=AND  UseBitMask=on  BitMask=bin2dec('0000000010000000000000000')  BitMaskRealWorld=Stored Integer
  Bitwise Operator13 : simulink/Logic and Bit Operations/Bitwise Operator  logicop=AND  UseBitMask=on  BitMask=bin2dec('0000000001000000000000000')  BitMaskRealWorld=Stored Integer
  Bitwise Operator14 : simulink/Logic and Bit Operations/Bitwise Operator  logicop=AND  UseBitMask=on  BitMask=bin2dec('0000000000100000000000000')  BitMaskRealWorld=Stored Integer
  Bitwise Operator15 : simulink/Logic and Bit Operations/Bitwise Operator  logicop=AND  UseBitMask=on  BitMask=bin2dec('0000000000010000000000000')  BitMaskRealWorld=Stored Integer
  Bitwise Operator16 : simulink/Logic and Bit Operations/Bitwise Operator  logicop=AND  UseBitMask=on  BitMask=bin2dec('0000000000001000000000000')  BitMaskRealWorld=Stored Integer
  Bitwise Operator17 : simulink/Logic and Bit Operations/Bitwise Operator  logicop=AND  UseBitMask=on  BitMask=bin2dec('0000000000000100000000000')  BitMaskRealWorld=Stored Integer
  Bitwise Operator18 : simulink/Logic and Bit Operations/Bitwise Operator  logicop=AND  UseBitMask=on  BitMask=bin2dec('0000000000000010000000000')  BitMaskRealWorld=Stored Integer
  Bitwise Operator19 : simulink/Logic and Bit Operations/Bitwise Operator  logicop=AND  UseBitMask=on  BitMask=bin2dec('0000000000000001000000000')  BitMaskRealWorld=Stored Integer
  Bitwise Operator20 : simulink/Logic and Bit Operations/Bitwise Operator  logicop=AND  UseBitMask=on  BitMask=bin2dec('0000000000000000100000000')  BitMaskRealWorld=Stored Integer
  Bitwise Operator21 : simulink/Logic and Bit Operations/Bitwise Operator  logicop=AND  UseBitMask=on  BitMask=bin2dec('0000000000000000010000000')  BitMaskRealWorld=Stored Integer
  Bitwise Operator22 : simulink/Logic and Bit Operations/Bitwise Operator  logicop=AND  UseBitMask=on  BitMask=bin2dec('0000000000000000001000000')  BitMaskRealWorld=Stored Integer
  Bitwise Operator23 : simulink/Logic and Bit Operations/Bitwise Operator  logicop=AND  UseBitMask=on  BitMask=bin2dec('0000000000000000000100000')  BitMaskRealWorld=Stored Integer
  Bitwise Operator24 : simulink/Logic and Bit Operations/Bitwise Operator  logicop=AND  UseBitMask=on  BitMask=bin2dec('0000000000000000000010000')  BitMaskRealWorld=Stored Integer
  Bitwise Operator25 : simulink/Logic and Bit Operations/Bitwise Operator  logicop=AND  UseBitMask=on  BitMask=bin2dec('0000000000000000000001000')  BitMaskRealWorld=Stored Integer
  Bitwise Operator26 : simulink/Logic and Bit Operations/Bitwise Operator  logicop=AND  UseBitMask=on  BitMask=bin2dec('0000000000000000000000100')  BitMaskRealWorld=Stored Integer
  Bitwise Operator27 : simulink/Logic and Bit Operations/Bitwise Operator  logicop=AND  UseBitMask=on  BitMask=bin2dec('0000000000000000000000010')  BitMaskRealWorld=Stored Integer
  Bitwise Operator28 : simulink/Logic and Bit Operations/Bitwise Operator  logicop=AND  UseBitMask=on  BitMask=bin2dec('0000000000000000000000001')  BitMaskRealWorld=Stored Integer
  Bitwise Operator6 : simulink/Logic and Bit Operations/Bitwise Operator  logicop=AND  UseBitMask=on  BitMask=bin2dec('0010000000000000000000000')  BitMaskRealWorld=Stored Integer
  Bitwise Operator7 : simulink/Logic and Bit Operations/Bitwise Operator  logicop=AND  UseBitMask=on  BitMask=bin2dec('0001000000000000000000000')  BitMaskRealWorld=Stored Integer
  Bitwise Operator8 : simulink/Logic and Bit Operations/Bitwise Operator  logicop=AND  UseBitMask=on  BitMask=bin2dec('0000100000000000000000000')  BitMaskRealWorld=Stored Integer
  Bitwise Operator9 : simulink/Logic and Bit Operations/Bitwise Operator  logicop=AND  UseBitMask=on  BitMask=bin2dec('0000010000000000000000000')  BitMaskRealWorld=Stored Integer
  Compare To Zero{1..24} (24 alike) : simulink/Logic and Bit Operations/Compare To Zero  SystemSampleTime=-1  relop=>  LogicOutDataTypeMode=uint8  ZeroCross=off
  Constant{1,8,10,12,14,16,18,20,22,24,26,28,30,32,34,36,38,40,42,44,46,48,50,52} (24 alike) : Constant  Value=2
  Constant{2,11,13,15,17,19,21,23,25,27,29,31,33,35,37,39,41,43,45,47,49,51,53} (23 alike) : Constant
  Display{1..8} (8 alike) : Display
  Math Function{1..24} (24 alike) : Math  Operator=pow  SaturateOnIntegerOverflow=on
  Product{1..24} (24 alike) : Product  RndMeth=Zero
  Sum{1,5..26} (23 alike) : Sum  Inputs=|+-
  Sum27 : Sum  Inputs=|++++++++++++++++++++++++
  Out1 : Outport
  wires:
  Product1/1 -> Sum27/24, Display7/1
  Sum1/1 -> Sum5/1, Display8/1, Math Function2/2
  Constant2/1 -> Sum1/2
  Math Function1/1 -> Product1/1
  Compare To Zero1/1 -> Product1/2
  Bitwise Operator1/1 -> Compare To Zero1/1
  Constant1/1 -> Math Function1/1
  Sum27/1 -> Out1/1
  In2/1 -> Bitwise Operator1/1, Bitwise Operator28/1, Bitwise Operator27/1, Bitwise Operator26/1, Bitwise Operator25/1, Bitwise Operator24/1, Bitwise Operator23/1, Bitwise Operator22/1, Bitwise Operator21/1, Bitwise Operator20/1, Bitwise Operator19/1, Bitwise Operator18/1, Bitwise Operator17/1, Bitwise Operator16/1, Bitwise Operator15/1, Bitwise Operator14/1, Bitwise Operator13/1, Bitwise Operator12/1, Bitwise Operator11/1, Bitwise Operator10/1, Bitwise Operator9/1, Bitwise Operator8/1, Bitwise Operator7/1, Bitwise Operator6/1
  In1/1 -> Sum1/1, Math Function1/2
  Product24/1 -> Sum27/1
  Product23/1 -> Sum27/2
  Product22/1 -> Sum27/23
  Product21/1 -> Sum27/22
  Product20/1 -> Sum27/21
  Product19/1 -> Sum27/20
  Product18/1 -> Sum27/19
  Product17/1 -> Sum27/18
  Product16/1 -> Sum27/17
  Product15/1 -> Sum27/16
  Product14/1 -> Sum27/15
  Product13/1 -> Sum27/14
  Product12/1 -> Sum27/13
  Product11/1 -> Sum27/12
  Product10/1 -> Sum27/11
  Product9/1 -> Sum27/10
  Product8/1 -> Sum27/9
  Product7/1 -> Display6/1, Sum27/8
  Product6/1 -> Display4/1, Sum27/7
  Product5/1 -> Display3/1, Sum27/6
  Product4/1 -> Display2/1, Sum27/5
  Product3/1 -> Display1/1, Sum27/4
  Product2/1 -> Display5/1, Sum27/3
  Sum26/1 -> Math Function24/2
  Constant53/1 -> Sum26/2
  Math Function24/1 -> Product24/1
  Compare To Zero24/1 -> Product24/2
  Bitwise Operator28/1 -> Compare To Zero24/1
  Constant52/1 -> Math Function24/1
  Sum25/1 -> Sum26/1, Math Function23/2
  Constant51/1 -> Sum25/2
  Math Function23/1 -> Product23/1
  Compare To Zero23/1 -> Product23/2
  Bitwise Operator27/1 -> Compare To Zero23/1
  Constant50/1 -> Math Function23/1
  Sum24/1 -> Sum25/1, Math Function22/2
  Constant49/1 -> Sum24/2
  Math Function22/1 -> Product22/1
  Compare To Zero22/1 -> Product22/2
  Bitwise Operator26/1 -> Compare To Zero22/1
  Constant48/1 -> Math Function22/1
  Sum23/1 -> Sum24/1, Math Function21/2
  Constant47/1 -> Sum23/2
  Math Function21/1 -> Product21/1
  Compare To Zero21/1 -> Product21/2
  Bitwise Operator25/1 -> Compare To Zero21/1
  Constant46/1 -> Math Function21/1
  Sum22/1 -> Sum23/1, Math Function20/2
  Constant45/1 -> Sum22/2
  Math Function20/1 -> Product20/1
  Compare To Zero20/1 -> Product20/2
  Bitwise Operator24/1 -> Compare To Zero20/1
  Constant44/1 -> Math Function20/1
  Sum21/1 -> Sum22/1, Math Function19/2
  Constant43/1 -> Sum21/2
  Math Function19/1 -> Product19/1
  Compare To Zero19/1 -> Product19/2
  Bitwise Operator23/1 -> Compare To Zero19/1
  Constant42/1 -> Math Function19/1
  Sum20/1 -> Sum21/1, Math Function18/2
  Constant41/1 -> Sum20/2
  Math Function18/1 -> Product18/1
  Compare To Zero18/1 -> Product18/2
  Bitwise Operator22/1 -> Compare To Zero18/1
  Constant40/1 -> Math Function18/1
  Sum19/1 -> Sum20/1, Math Function17/2
  Constant39/1 -> Sum19/2
  Math Function17/1 -> Product17/1
  Compare To Zero17/1 -> Product17/2
  Bitwise Operator21/1 -> Compare To Zero17/1
  Constant38/1 -> Math Function17/1
  Sum18/1 -> Sum19/1, Math Function16/2
  Constant37/1 -> Sum18/2
  Math Function16/1 -> Product16/1
  Compare To Zero16/1 -> Product16/2
  Bitwise Operator20/1 -> Compare To Zero16/1
  Constant36/1 -> Math Function16/1
  Sum17/1 -> Sum18/1, Math Function15/2
  Constant35/1 -> Sum17/2
  Math Function15/1 -> Product15/1
  Compare To Zero15/1 -> Product15/2
  Bitwise Operator19/1 -> Compare To Zero15/1
  Constant34/1 -> Math Function15/1
  Sum16/1 -> Sum17/1, Math Function14/2
  Constant33/1 -> Sum16/2
  Math Function14/1 -> Product14/1
  Compare To Zero14/1 -> Product14/2
  Bitwise Operator18/1 -> Compare To Zero14/1
  Constant32/1 -> Math Function14/1
  Sum15/1 -> Sum16/1, Math Function13/2
  Constant31/1 -> Sum15/2
  Math Function13/1 -> Product13/1
  Compare To Zero13/1 -> Product13/2
  Bitwise Operator17/1 -> Compare To Zero13/1
  Constant30/1 -> Math Function13/1
  Sum14/1 -> Sum15/1, Math Function12/2
  Constant29/1 -> Sum14/2
  Math Function12/1 -> Product12/1
  Compare To Zero12/1 -> Product12/2
  Bitwise Operator16/1 -> Compare To Zero12/1
  Constant28/1 -> Math Function12/1
  Sum13/1 -> Sum14/1, Math Function11/2
  Constant27/1 -> Sum13/2
  Math Function11/1 -> Product11/1
  Compare To Zero11/1 -> Product11/2
  Bitwise Operator15/1 -> Compare To Zero11/1
  Constant26/1 -> Math Function11/1
  Sum12/1 -> Sum13/1, Math Function10/2
  Constant25/1 -> Sum12/2
  Math Function10/1 -> Product10/1
  Compare To Zero10/1 -> Product10/2
  Bitwise Operator14/1 -> Compare To Zero10/1
  Constant24/1 -> Math Function10/1
  Sum11/1 -> Sum12/1, Math Function9/2
  Constant23/1 -> Sum11/2
  Math Function9/1 -> Product9/1
  Compare To Zero9/1 -> Product9/2
  Bitwise Operator13/1 -> Compare To Zero9/1
  Constant22/1 -> Math Function9/1
  Sum10/1 -> Sum11/1, Math Function8/2
  Constant21/1 -> Sum10/2
  Math Function8/1 -> Product8/1
  Compare To Zero8/1 -> Product8/2
  Bitwise Operator12/1 -> Compare To Zero8/1
  Constant20/1 -> Math Function8/1
  Sum9/1 -> Sum10/1, Math Function7/2
  Constant19/1 -> Sum9/2
  Math Function7/1 -> Product7/1
  Compare To Zero7/1 -> Product7/2
  Bitwise Operator11/1 -> Compare To Zero7/1
  Constant18/1 -> Math Function7/1
  Sum8/1 -> Math Function6/2, Sum9/1
  Constant17/1 -> Sum8/2
  Math Function6/1 -> Product6/1
  Compare To Zero6/1 -> Product6/2
  Bitwise Operator10/1 -> Compare To Zero6/1
  Constant16/1 -> Math Function6/1
  Sum7/1 -> Math Function5/2, Sum8/1
  Constant15/1 -> Sum7/2
  Math Function5/1 -> Product5/1
  Compare To Zero5/1 -> Product5/2
  Bitwise Operator9/1 -> Compare To Zero5/1
  Constant14/1 -> Math Function5/1
  Sum6/1 -> Math Function4/2, Sum7/1
  Constant13/1 -> Sum6/2
  Math Function4/1 -> Product4/1
  Compare To Zero4/1 -> Product4/2
  Bitwise Operator8/1 -> Compare To Zero4/1
  Constant12/1 -> Math Function4/1
  Sum5/1 -> Math Function3/2, Sum6/1
  Constant11/1 -> Sum5/2
  Math Function3/1 -> Product3/1
  Compare To Zero3/1 -> Product3/2
  Bitwise Operator7/1 -> Compare To Zero3/1
  Constant10/1 -> Math Function3/1
  Math Function2/1 -> Product2/1
  Compare To Zero2/1 -> Product2/2
  Bitwise Operator6/1 -> Compare To Zero2/1
  Constant8/1 -> Math Function2/1
